simulink model "heli_q8"  (R2020b)
settings: Solver=ode1  StartTime=0.0  StopTime=inf  FixedStep=0.002  RelTol=1e-3  EnableMultiTasking=on
PostLoadFcn:
  | qc_set_target_type(getConfigSet(bdroot, 'QUARC Default Target Configuration'));
values from neighbouring files (symbols this model uses):
  e_0 = 0.528    [init_heli_3_10.m]
  F = [K(1,1), K(1,3); K(2,1), K(2,3)]    [init_heli_3_10.m]
  Joystick_gain_x = 1    [init_heli_3_10.m]
  Joystick_gain_y = -1    [init_heli_3_10.m]
  K = place(A, B, poles_des)    [init_heli_3_10.m]
  P = 0.175    [init_heli_3_10.m]
  sw_ecdot = 2    [init_heli_3_10.m]
  sw_pc = 2    [init_heli_3_10.m]
  t1 = 20    [init_heli_3_10.m]
  t2 = 23    [init_heli_3_10.m]
  t3 = 24    [init_heli_3_10.m]
  t4 = 26    [init_heli_3_10.m]
  Vs_0 = 7    [init_heli_3_10.m]
undefined symbols (not defined in the file or in its folder): HIL, qc_get_step_size
libraries: quarc_library x4
settings Model: SimulationMode=external  ExtModeBatchMode=on  ExtModeTrigDuration=30000  Creator=Rchan  LastModifiedBy=alpery
settings SolverCC: PositivePriorityOrder=on
settings DataIOCC: LimitDataPoints=on  SaveFormat=Array  SignalLoggingSaveFormat=ModelDataLogs  ReturnWorkspaceOutputs=off
settings OptimizationCC: ExpressionDepthLimit=2147483647  InitFltsAndDblsToZero=on  LifeSpan=inf
settings DebuggingCC: SaveWithParameterizedLinksMsg=none  UnderspecifiedInitializationDetection=Classic  MergeDetectMultiDrivingBlocksExec=none  SolverPrmCheckMsg=warning  MultiTaskDSMMsg=warning  MultiTaskCondExecSysMsg=none  FcnCallInpInsideContextMsg=warning  AllowSymbolicDim=off  StateNameClashWarn=warning  SFUnexpectedBacktrackingDiag=warning  SFNoUnconditionalDefaultTransitionDiag=warning  SFExecutionAtInitializationDiag=none  ArithmeticOperatorsInVariantConditions=warning
settings HardwareCC: ProdBitPerPointer=32  ProdBitPerSizeT=32  ProdBitPerPtrDiffT=32  ProdLargestAtomicFloat=None  ProdIntDivRoundTo=Undefined  ProdEndianess=Unspecified  ProdWordSize=32  ProdHWDeviceType=32-bit Generic
settings ModelReferenceCC: PropagateSignalLabelsOutOfModel=off
settings SFSimCC: SimUseLocalCustomCode=off  CustomCodeUndefinedFunction=UseInterfaceOnly
settings RTWCC: Description=QUARC Win64 Target  SystemTargetFile=quarc_win64.tlc  TemplateMakefile=quarc_default_tmf  RTWUseLocalCustomCode=off
settings CodeAppCC: StateflowObjectComments=on
settings GRTTargetCC: TargetLangStandard=C89/C90 (ANSI)  ParMdlRefBuildCompliant=off  CompOptLevelCompliant=off  CombineOutputUpdateFcns=off  MatFileLogging=off  GRTInterface=on  UseToolchainInfoCompliant=off  ExtMode=on  ExtModeMexFile=quarc_comm
settings ConfigComp: CovMetricSettings=dw  CovSaveCumulativeToWorkspaceVar=on  CovSaveSingleToWorkspaceVar=on  CovExternalEMLEnable=off  CovSFcnEnable=off

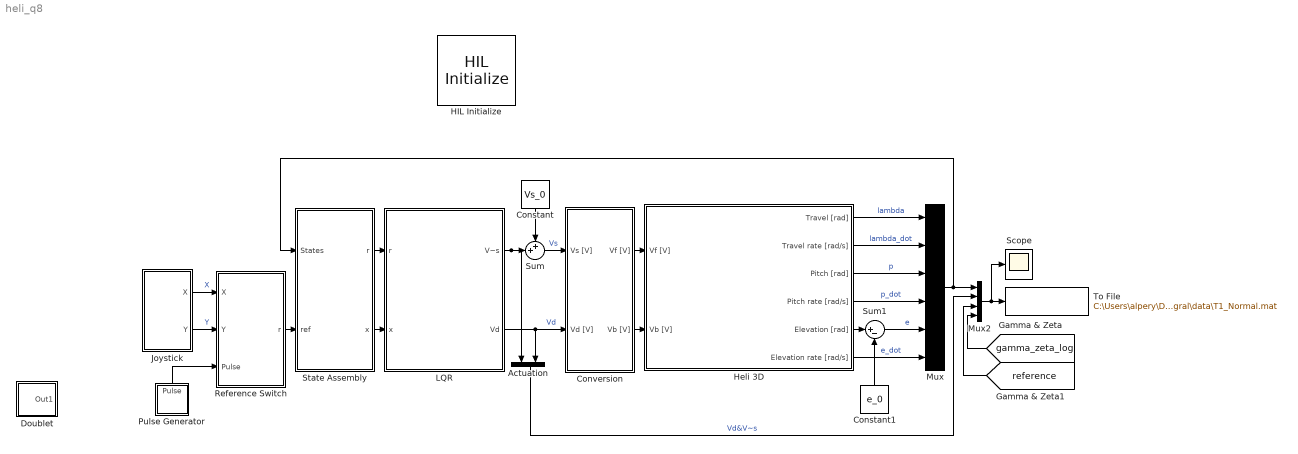
== system heli_q8 ==
  Actuation : Mux  Inputs=2
  Constant : Constant  Value=Vs_0
  Constant1 : Constant  Value=e_0
  Conversion : Subsystem
  Doublet : Subsystem
  HIL Initialize : quarc_library/Data Acquisition/Generic/Configuration/HIL Initialize  Priority=-99  object_name=HIL-1  board_type=q8_usb  board_number=0  board_options=update_rate=normal;decimation=1  exclusive=off  active=off  hardware_clocks=[0:2]  clock_modes=[]  initial_clock_frequencies=[]  set_clock_params_at_start=off  set_clock_params_at_switch_in=off  set_clock_frequencies_at_start=off  set_clock_frequencies_at_switch_in=off  analog_input_channels=[0:7]  analog_input_configurations=[]  analog_input_maximums=10  analog_input_minimums=-10  set_analog_input_params_at_start=on  set_analog_input_params_at_switch_in=off  analog_output_channels=[0:7]  analog_output_maximums=10  analog_output_minimums=-10  initial_analog_outputs=[0]  final_analog_outputs=[0]  watchdog_analog_outputs=0  set_analog_output_params_at_start=on  set_analog_output_params_at_switch_in=off  set_analog_outputs_at_start=on  set_analog_outputs_at_switch_in=off  set_analog_outputs_at_terminate=on  set_analog_outputs_at_switch_out=off  set_analog_outputs_on_watchdog=off  digital_input_channels=[]  digital_output_channels=[]  digital_output_configuration=[]  initial_digital_outputs=[1]  final_digital_outputs=[1]  watchdog_digital_outputs=[1]  set_digital_output_params_at_start=off  set_digital_output_params_at_switch_in=off  set_digital_outputs_at_start=on  set_digital_outputs_at_switch_in=off  set_digital_outputs_at_terminate=on  set_digital_outputs_at_switch_out=off  set_digital_outputs_on_watchdog=off  encoder_channels=[0:7]  quadrature=[4]  encoder_filter_frequency=[]  initial_encoder_counts=[0]  set_encoder_params_at_start=on  set_encoder_params_at_switch_in=off  set_encoder_counts_at_start=on  set_encoder_counts_at_switch_in=off  pwm_channels=[0:7]  pwm_modes=0  pwm_frequency=99.532799999999995e6/4095  pwm_configuration=[0]  pwm_alignment=[0]  pwm_polarity=[1]  pwm_leading_deadband=[0]  pwm_trailing_deadband=[0]  initial_pwm_outputs=[0]  final_pwm_outputs=[0]  watchdog_pwm_outputs=[0]  set_pwm_params_at_start=on  set_pwm_params_at_switch_in=off  set_pwm_outputs_at_start=on  set_pwm_outputs_at_switch_in=off  set_pwm_outputs_at_terminate=on  set_pwm_outputs_at_switch_out=off  set_pwm_outputs_on_watchdog=off  other_output_channels=[]  initial_other_outputs=[]  final_other_outputs=[]  watchdog_other_outputs=[]  set_other_outputs_at_start=off  set_other_outputs_at_switch_in=off  set_other_outputs_at_terminate=off  set_other_outputs_at_switch_out=off  set_other_outputs_on_watchdog=off
  Heli 3D : Subsystem
  Joystick : Subsystem
  LQR : Subsystem
  Mux : Mux  Inputs=6
  Mux2 : Mux
  Pulse Generator : Subsystem
  Reference Switch : Subsystem
  Scope : Scope
  State Assembly : Subsystem
  Sum : Sum  Inputs=++|
  Sum1 : Sum  Inputs=|+-
  To File : ToFile  Filename=C:\Users\alpery\Documents\Helikopter\Task 2.2 - LQR w Integral\data\T1_Normal.mat  MatrixName=heli_log
  wires:
  Conversion/2(Vb [V]) -> Heli 3D/2(Vb [V])
  Conversion/1(Vf [V]) -> Heli 3D/1(Vf [V])
  Heli 3D/1(Travel [rad]) -> Mux/1  "lambda"
  Heli 3D/2(Travel rate [rad/s]) -> Mux/2  "lambda_dot"
  Heli 3D/4(Pitch rate [rad/s]) -> Mux/4  "p_dot"
  Heli 3D/6(Elevation rate [rad/s]) -> Mux/6  "e_dot"
  Sum/1 -> Conversion/1(Vs [V])  "Vs"
  Heli 3D/5(Elevation [rad]) -> Sum1/1
  Sum1/1 -> Mux/5  "e"
  Constant1/1 -> Sum1/2
  Heli 3D/3(Pitch [rad]) -> Mux/3  "p"
  Constant/1 -> Sum/1
  LQR/1(V~s) -> Actuation/1, Sum/2
  State Assembly/1(r) -> LQR/1(r)
  LQR/2(Vd) -> Actuation/2, Conversion/2(Vd [V])  "Vd"
  Mux/1 -> Mux2/1, State Assembly/1(States)
  State Assembly/2(x) -> LQR/2(x)
  Joystick/2(Y) -> Reference Switch/2(Y)  "Y"
  Mux2/1 -> Scope/1, To File/1
  Actuation/1 -> Mux2/2  "Vd&V~s"
  Reference Switch/1(r) -> State Assembly/2(ref)
  Joystick/1(X) -> Reference Switch/1(X)  "X"
  [reference] -> Mux2/3
  [gamma_zeta_log] -> Mux2/4
  Pulse Generator/1(Pulse) -> Reference Switch/3(Pulse)

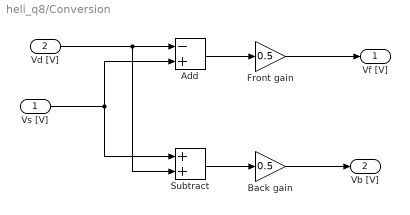
== system heli_q8/Conversion ==
  Vs [V] : Inport
  Vd [V] : Inport  Port=2
  Add : Sum  Inputs=-+
  Back gain : Gain  Gain=0.5
  Front gain : Gain  Gain=0.5
  Subtract : Sum
  Vf [V] : Outport
  Vb [V] : Outport  Port=2
  wires:
  Vd [V]/1 -> Subtract/2, Add/1
  Vs [V]/1 -> Subtract/1, Add/2
  Subtract/1 -> Back gain/1
  Back gain/1 -> Vb [V]/1
  Add/1 -> Front gain/1
  Front gain/1 -> Vf [V]/1

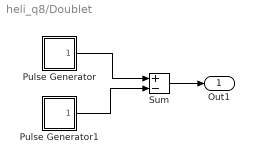
== system heli_q8/Doublet ==
  Pulse Generator : Subsystem
  Pulse Generator1 : Subsystem
  Sum : Sum  Inputs=+-
  Out1 : Outport
  wires:
  Sum/1 -> Out1/1
  Pulse Generator/1(Pulse) -> Sum/1
  Pulse Generator1/1(Pulse) -> Sum/2

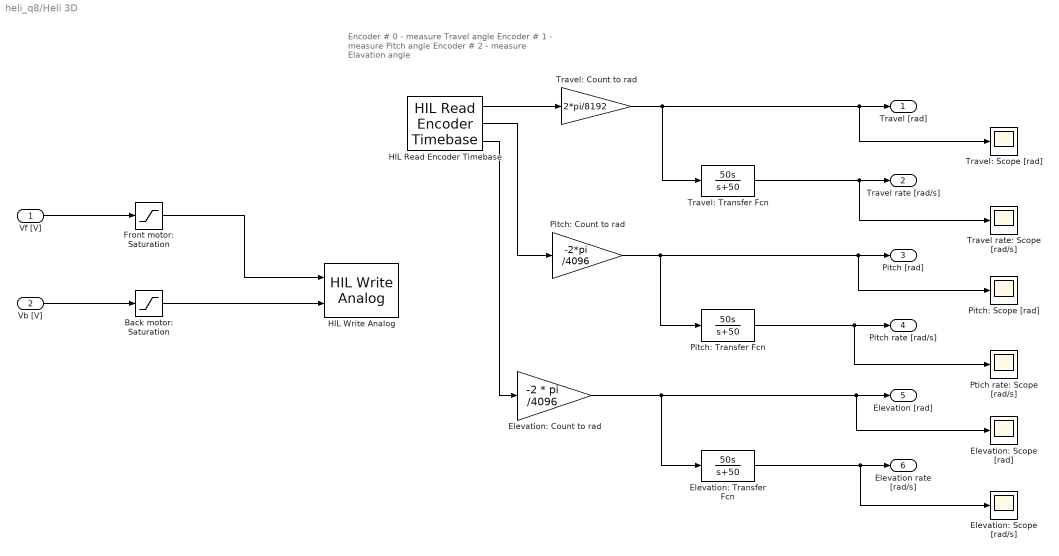
== system heli_q8/Heli 3D ==
  note: Encoder # 0 - measure Travel angle
      | Encoder # 1 - measure Pitch angle
      | Encoder # 2 - measure Elavation angle
  Vf [V] : Inport
  Vb [V] : Inport  Port=2
  Back motor: Saturation : Saturate  UpperLimit=5  LowerLimit=-5
  Elevation: Count to rad : Gain  Gain=-2 * pi /4096
  Elevation: Scope [rad/s] : Scope
  Elevation: Scope [rad] : Scope
  Elevation: Transfer Fcn : TransferFcn  Numerator=[50 0]  Denominator=[1 50]
  Front motor: Saturation : Saturate  UpperLimit=5  LowerLimit=-5
  HIL Read Encoder Timebase : quarc_library/Data Acquisition/Generic/Timebases/HIL Read Encoder Timebase  object_name=HIL-1  clock=0  channels=[0:2]  active=on  vector_output=off  data_type_mode=Inherit via back propagation  data_type=double  overflow_mode=Error on overflow  samples_in_buffer=max(ceil(1/qc_get_step_size), 1)
  HIL Write Analog : quarc_library/Data Acquisition/Generic/Immediate I//O/HIL Write Analog  object_name=HIL-1  channels=[0:1]  sample_time=-1  active=off  vector_input=off
  Pitch: Count to rad : Gain  Gain=-2*pi /4096
  Pitch: Scope [rad] : Scope
  Pitch: Transfer Fcn : TransferFcn  Numerator=[50 0]  Denominator=[1 50]
  Ptich rate: Scope [rad/s] : Scope
  Travel rate: Scope [rad/s] : Scope
  Travel: Count to rad : Gain  Gain=2*pi/8192
  Travel: Scope [rad] : Scope
  Travel: Transfer Fcn : TransferFcn  Numerator=[50 0]  Denominator=[1 50]
  Travel [rad] : Outport
  Travel rate [rad/s] : Outport  Port=2
  Pitch [rad] : Outport  Port=3
  Pitch rate [rad/s] : Outport  Port=4
  Elevation [rad] : Outport  Port=5
  Elevation rate [rad/s] : Outport  Port=6
  wires:
  HIL Read Encoder Timebase/1 -> Travel: Count to rad/1
  HIL Read Encoder Timebase/2 -> Pitch: Count to rad/1
  HIL Read Encoder Timebase/3 -> Elevation: Count to rad/1
  Travel: Count to rad/1 -> Travel: Scope [rad]/1, Travel [rad]/1, Travel: Transfer Fcn/1
  Travel: Transfer Fcn/1 -> Travel rate: Scope [rad/s]/1, Travel rate [rad/s]/1
  Pitch: Count to rad/1 -> Pitch: Transfer Fcn/1, Pitch: Scope [rad]/1, Pitch [rad]/1
  Pitch: Transfer Fcn/1 -> Ptich rate: Scope [rad/s]/1, Pitch rate [rad/s]/1
  Elevation: Count to rad/1 -> Elevation: Transfer Fcn/1, Elevation: Scope [rad]/1, Elevation [rad]/1
  Elevation: Transfer Fcn/1 -> Elevation: Scope [rad/s]/1, Elevation rate [rad/s]/1
  Vf [V]/1 -> Front motor: Saturation/1
  Vb [V]/1 -> Back motor: Saturation/1
  Front motor: Saturation/1 -> HIL Write Analog/1
  Back motor: Saturation/1 -> HIL Write Analog/2

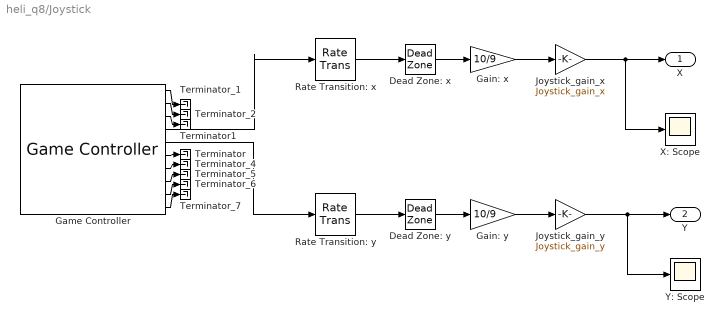
== system heli_q8/Joystick ==
  Dead Zone: x : DeadZone  LowerValue=-0.1  UpperValue=0.1  SaturateOnIntegerOverflow=on
  Dead Zone: y : DeadZone  LowerValue=-0.1  UpperValue=0.1  SaturateOnIntegerOverflow=on
  Gain: x : Gain  Gain=10/9
  Gain: y : Gain  Gain=10/9
  Game Controller : quarc_library/Devices/Peripherals/Target/Game Controller  controller=1  buffer_size=12  deadzone=[]  saturation=[]  sample_time=max(qc_get_step_size, 0.01)  auto_center=off  enabled=on
      settings: SourceProductName=QUARC Targets
  Joystick_gain_x : Gain  Gain=Joystick_gain_x
  Joystick_gain_y : Gain  Gain=Joystick_gain_y
  Rate Transition: x : RateTransition
  Rate Transition: y : RateTransition
  Terminator : Terminator
  Terminator1 : Terminator
  Terminator_{1..2,4..7} (6 alike) : Terminator
  X: Scope : Scope
  Y: Scope : Scope
  X : Outport
  Y : Outport  Port=2
  wires:
  Rate Transition: y/1 -> Dead Zone: y/1
  Rate Transition: x/1 -> Dead Zone: x/1
  Game Controller/5 -> Rate Transition: y/1
  Game Controller/4 -> Rate Transition: x/1
  Game Controller/1 -> Terminator_1/1
  Game Controller/2 -> Terminator_2/1
  Game Controller/7 -> Terminator_4/1
  Game Controller/8 -> Terminator_5/1
  Game Controller/9 -> Terminator_6/1
  Game Controller/10 -> Terminator_7/1
  Game Controller/3 -> Terminator1/1
  Game Controller/6 -> Terminator/1
  Dead Zone: x/1 -> Gain: x/1
  Dead Zone: y/1 -> Gain: y/1
  Gain: x/1 -> Joystick_gain_x/1
  Gain: y/1 -> Joystick_gain_y/1
  Joystick_gain_x/1 -> X/1, X: Scope/1
  Joystick_gain_y/1 -> Y: Scope/1, Y/1

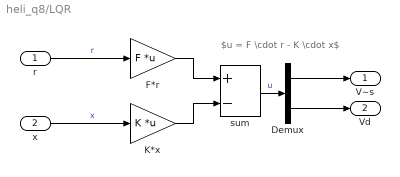
== system heli_q8/LQR ==
  note: $u = F \cdot r - K \cdot x$
  r : Inport
  x : Inport  Port=2
  Demux : Demux  Outputs=2
  F*r : Gain  Gain=F  Multiplication=Matrix(K*u)
  K*x : Gain  Gain=K  Multiplication=Matrix(K*u)
  sum : Sum  Inputs=+-
  V~s : Outport
  Vd : Outport  Port=2
  wires:
  r/1 -> F*r/1  "r"
  F*r/1 -> sum/1
  K*x/1 -> sum/2
  sum/1 -> Demux/1  "u"
  Demux/1 -> V~s/1
  Demux/2 -> Vd/1
  x/1 -> K*x/1  "x"

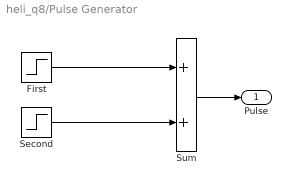
== system heli_q8/Pulse Generator ==
  First : Step  Time=t1  After=P  SampleTime=0
  Second : Step  Time=t2  After=-P  SampleTime=0
  Sum : Sum
  Pulse : Outport
  wires:
  Sum/1 -> Pulse/1
  Second/1 -> Sum/2
  First/1 -> Sum/1

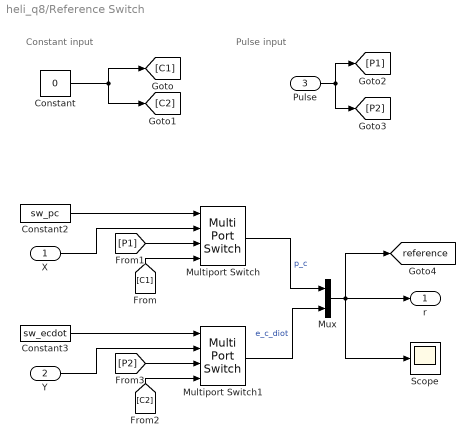
== system heli_q8/Reference Switch ==
  note: Pulse input
  note: Constant input
  X : Inport
  Y : Inport  Port=2
  Pulse : Inport  Port=3
  Constant : Constant  Value=0
  Constant2 : Constant  Value=sw_pc
  Constant3 : Constant  Value=sw_ecdot
  Multiport Switch : MultiPortSwitch
  Multiport Switch1 : MultiPortSwitch
  Mux : Mux  Inputs=2
  Scope : Scope
  r : Outport
  tag scope: reference=global
  wires:
  Mux/1 -> Scope/1, r/1, [reference]
  Multiport Switch/1 -> Mux/1  "p_c"
  X/1 -> Multiport Switch/2
  Constant/1 -> [C2], [C1]
  Pulse/1 -> [P2], [P1]
  [C1] -> Multiport Switch/4
  [P1] -> Multiport Switch/3
  [P2] -> Multiport Switch1/3
  Constant3/1 -> Multiport Switch1/1
  Y/1 -> Multiport Switch1/2
  [C2] -> Multiport Switch1/4
  Multiport Switch1/1 -> Mux/2  "e_c_diot"
  Constant2/1 -> Multiport Switch/1

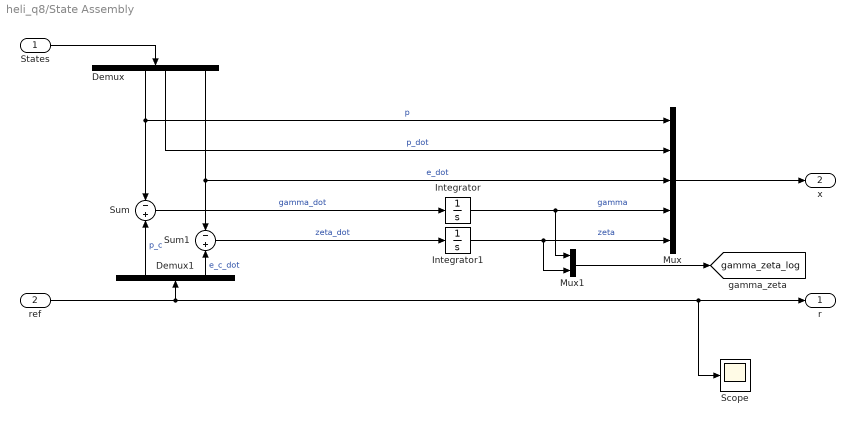
== system heli_q8/State Assembly ==
  States : Inport
  ref : Inport  Port=2
  Demux : Demux  Outputs=6
  Demux1 : Demux  Outputs=2
  Integrator : Integrator
  Integrator1 : Integrator  InitialCondition=e_0
  Mux : Mux  Inputs=5
  Mux1 : Mux  Inputs=2
  Scope : Scope
  Sum : Sum  Inputs=-|+
  Sum1 : Sum  Inputs=-|+
  r : Outport
  x : Outport  Port=2
  tag scope: gamma_zeta_log=global
  wires:
  States/1 -> Demux/1
  ref/1 -> Scope/1, r/1, Demux1/1
  Demux1/1 -> Sum/2  "p_c"
  Demux/3 -> Mux/1, Sum/1  "p"
  Sum/1 -> Integrator/1  "gamma_dot"
  Demux1/2 -> Sum1/2  "e_c_dot"
  Demux/6 -> Mux/3, Sum1/1  "e_dot"
  Sum1/1 -> Integrator1/1  "zeta_dot"
  Mux/1 -> x/1
  Integrator1/1 -> Mux1/2, Mux/5  "zeta"
  Integrator/1 -> Mux1/1, Mux/4  "gamma"
  Demux/4 -> Mux/2  "p_dot"
  Mux1/1 -> [gamma_zeta_log]

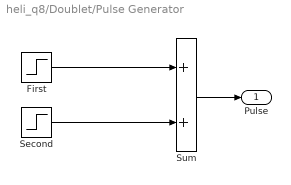
== system heli_q8/Doublet/Pulse Generator ==
  First : Step  Time=t1  After=P  SampleTime=0
  Second : Step  Time=t2  After=-P  SampleTime=0
  Sum : Sum
  Pulse : Outport
  wires:
  Sum/1 -> Pulse/1
  Second/1 -> Sum/2
  First/1 -> Sum/1

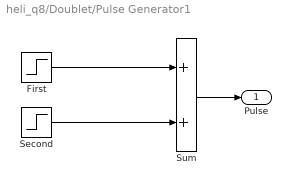
== system heli_q8/Doublet/Pulse Generator1 ==
  First : Step  Time=t3  After=P  SampleTime=0
  Second : Step  Time=t4  After=-P  SampleTime=0
  Sum : Sum
  Pulse : Outport
  wires:
  Sum/1 -> Pulse/1
  Second/1 -> Sum/2
  First/1 -> Sum/1
